simulink model "ROSPiNav2"  (Simulink 10.0)
settings: Solver=FixedStepAuto  StartTime=0.0  StopTime=inf  RelTol=1e-3
libraries: sensehatlib x5, robotlib x2, simulink x1, raspberrypilib x1
settings Model: LogicAnalyzerSignalOrdering=0b4ee2b6-c9ba-4ba2-86b4-30ad931c7907,c8c877dd-a2d7-4449-817a-3d091eaa01f0,b65482df-6083-4df0-8804-932ee4a1c904,d5d3a0d7-9de6-498d-bd3e-b3a3d3b67ba2,3bc10de9-2fa7-4451-9b63-790e2e79518c  Creator=FRED-Surface  LastModifiedBy=FRED-Surface
settings Model: SuppressorTable=|
  | <?xml version="1.0" encoding="UTF-8" standalone="yes" ?>
  | <!DOCTYPE boost_serialization>
  | <boost_serialization signature="serialization::archive" version="15">
  | <DiagnosticSuppressor class_id="0" tracking_level="0" version="6">
  | 	<Table class_id="1" tracking_level="0" version="0">
  | 		<count>1</count>
  | 		<bucket_count>8</bucket_count>
  | 		<item_version>0</item_version>
  | 		<item class_id="2" tracking_level="0" version="0">
  | 			<first class_id="3" tracking_level="0" version="6">
  | 				<Source class_id="4" tracking_level="0" version="0">
  | 					<count>1</count>
  | 					<item_version>0</item_version>
  | 					<item>ROSPiNav2/Counter Limited</item>
  | 				</Source>
  | 			</first>
  | 			<second class_id="5" tracking_level="0" version="6">
  | 				<SuppressedData class_id="6" tracking_level="0" version="0">
  | 					<count>2</count>
  | 					<bucket_count>8</bucket_count>
  | 					<item_version>0</item_version>
  | 					<item class_id="7" tracking_level="0" version="0">
  | 						<first class_id="8" tracking_level="0" version="6">
  | 							<ID>Simulink:DataType:WarningOverFlowDetected</ID>
  | 							<Cause>
  | 								<Source>
  | 									<count>0</count>
  | 									<item_version>0</item_version>
  | 								</Source>
  | 							</Cause>
  | 						</first>
  | 						<second class_id="9" tracking_level="0" version="6">
  | 							<Comment></Comment>
  | 							<User></User>
  | 							<LastModified class_id="10" tracking_level="0" version="0">
  | 								<ptime_date class_id="11" tracking_level="0" version="0">
  | 									<date>20160608</date>
  | 								</ptime_date>
  | 								<ptime_time_duration class_id="12" tracking_level="0" version="0">
  | 									<is_special>0</is_special>
  | 									<time_duration_hours>15</time_duration_hours>
  | 									<time_duration_minutes>23</time_duration_minutes>
  | 									<time_duration_seconds>17</time_duration_seconds>
  | 									<time_duration_fractional_seconds>0</time_duration_fractional_seconds>
  | 								</ptime_time_duration>
  | 							</LastModified>
  | 							<SuppressionType>1</SuppressionType>
  | 						</second>
  | 					</item>
  | 					<item>
  | 						<first>
  | 							<ID>SimulinkFixedPoint:util:Overflowoccurred</ID>
  | 							<Cause>
  | 								<Source>
  | 									<count>0</count>
  | 									<item_version>0</item_version>
  | 								</Source>
  | 							</Cause>
  | 						</first>
  | 						<second>
  | 							<Comment></Comment>
  | 							<User></User>
  | 							<LastModified>
  | 								<ptime_date>
  | 									<date>20160608</date>
  | 								</ptime_date>
  | 								<ptime_time_duration>
  | 									<is_special>0</is_special>
  | 									<time_duration_hours>15</time_duration_hours>
  | 									<time_duration_minutes>23</time_duration_minutes>
  | 									<time_duration_seconds>17</time_duration_seconds>
  | 									<time_duration_fractional_seconds>0</time_duration_fractional_seconds>
  | 								</ptime_time_duration>
  | 							</LastModified>
  | 							<SuppressionType>1</SuppressionType>
  | 						</second>
  | 					</item>
  | 				</SuppressedData>
  | 			</second>
  | 		</item>
  | 	</Table>
  | </DiagnosticSuppressor>
  | </boost_serialization>
settings DataIOCC: SaveFormat=Dataset  ReturnWorkspaceOutputs=on
settings OptimizationCC: EnhancedBackFolding=on  PassReuseOutputArgsAs=Individual arguments  ZeroExternalMemoryAtStartup=off  ZeroInternalMemoryAtStartup=off  LifeSpan=auto  MaxStackSize=64  OptimizeBlockOrder=speed  DifferentSizesBufferReuse=on  OptimizationCustomize=off  EfficientTunableParamExpr=on
settings DebuggingCC: UnderspecifiedInitializationDetection=Simplified  MergeDetectMultiDrivingBlocksExec=error  ParameterTunabilityLossMsg=error  SFUnexpectedBacktrackingDiag=error  SFNoUnconditionalDefaultTransitionDiag=error  SFExecutionAtInitializationDiag=warning  ArithmeticOperatorsInVariantConditions=error
settings HardwareCC: ProdLargestAtomicInteger=Long  ProdLargestAtomicFloat=Double  ProdIntDivRoundTo=Zero  ProdEndianess=LittleEndian  ProdHWDeviceType=ARM Compatible->ARM Cortex
settings ModelReferenceCC: PropagateSignalLabelsOutOfModel=on
settings SFSimCC: SimUseLocalCustomCode=on  MATLABDynamicMemAlloc=off  CustomCodeUndefinedFunction=FilterOut
settings RTWCC: Description=Embedded Coder  SystemTargetFile=ert.tlc  HardwareBoard=Robot Operating System (ROS)  TLCOptions="-aInlineSetEventsForThisBaseRateFcn=TLC_FALSE -aSuppressMultiTaskScheduler=TLC_FALSE  -aRateBasedStepFcn=0"  TemplateMakefile=ert_default_tmf  GenerateReport=on  RTWUseLocalCustomCode=on  Toolchain=Catkin  IncludeHyperlinkInReport=on  LaunchReport=on  TargetLang=C++  GenerateTraceInfo=on  GenerateTraceReport=on  GenerateTraceReportSl=on  GenerateTraceReportSf=on  GenerateTraceReportEml=on
settings MATStruct: className=codertarget.tools.BuildHook  argsTopModelOnly=[]  excludedModels=[]  includeReferencedModels=on  includeTopModel=on  enabled=on  UseCoderTarget=[1]  TargetHardware=Robot Operating System (ROS)  RTOS=Linux  RTOSBaseRateTaskPriority=40  DetectTaskOverruns=[0.0]  Scheduler_interrupt_source=[0.0]  DataVersion=2016.02  IPAddress=ros.codertarget.internal.DeviceParameters.getDeviceAddress  Port=17725  Verbose=[0]  RunInBackground=[1]  Configuration=TCP/IP  MaintainerName=ROS User  MaintainerEmail=rosuser@test.com  License=BSD  DeviceAddress=192.168.0.102  Username=ubuntu  BuildAction=None  Install=/opt/ros/melodic  CatkinWS=~/catkin_ws  ROSTimeStepping=0  ROSTimeNotification=0  StepNotify=/step_notify
settings CodeAppCC: ForceParamTrailComments=on  IgnoreCustomStorageClasses=off  OperatorAnnotations=on  SimulinkDataObjDesc=on  SFDataObjDesc=on  InsertBlockDesc=on  StateflowObjectComments=off
settings ConfigComp: CovMetricSettings=dwe  CovHtmlReporting=off  CovSaveCumulativeToWorkspaceVar=off  CovSaveSingleToWorkspaceVar=off

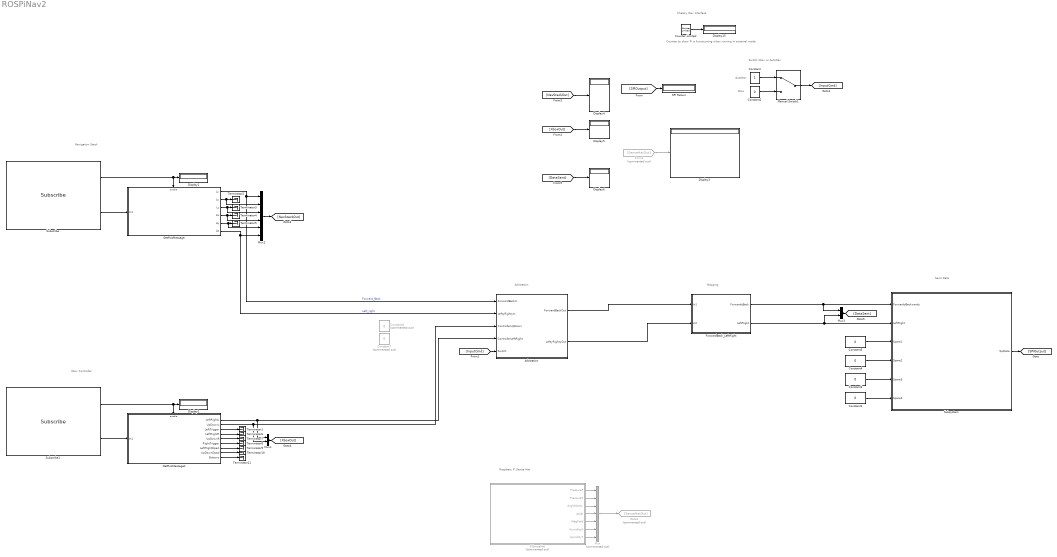
== system ROSPiNav2 ==
  note: Arbitration
  note: Xbox Controller
  note: Raspbery Pi Sense Hat
  note: Switch Xbox or AutoNav
  note: Cheeky Dev Interface
  note: Xbox
  note: Counter to show Pi is functiuoning when running in external mode
  note: Send Data
  note: Navigation Stack
  note: Mapping
  note: AutoNav
  Arbitration : Subsystem
  Constant : Constant  OutDataTypeStr=single
  Constant{1..5} (5 alike) : Constant  Value=0  OutDataTypeStr=single
  Constant6 : Constant  Commented=on  Value=0  OutDataTypeStr=single
  Constant7 : Constant  Commented=on  Value=0  OutDataTypeStr=single
  Counter Limited : simulink/Sources/Counter Limited  uplimit=7  tsamp=1
  Display{1..6,15} (7 alike) : Display
      Display15 settings: Format=bank  Decimation=2
      Display3 settings: Format=bank  Decimation=2
  ForwardBack_LeftRight : Subsystem
  From2 : From  Commented=on  GotoTag=SenseHatOut
  GetRosMessage : Subsystem
  GetRosMessage1 : Subsystem
  Goto2 : Goto  Commented=on  GotoTag=SenseHatOut
  Manual Switch1 : ManualSwitch
  Mux : Mux  Commented=on  Inputs=7
  Mux1 : Mux  Inputs=2
  Mux2 : Mux  Inputs=6
  Mux3 : Mux  Inputs=2
  PiSenseHat : Subsystem  Commented=on
  SPI Return : Display
      settings: Format=bank  Decimation=2
  Subscribe : robotlib/Subscribe  topicSource=Select from ROS network  topic=/planner/cmd_vel  messageType=geometry_msgs/Twist  sampleTime=0.1  messageQueueLength=1
      settings: SourceProductName=ROS Toolbox
  Subscribe1 : robotlib/Subscribe  topicSource=Specify your own  topic=/joy  messageType=sensor_msgs/Joy  sampleTime=0.1  messageQueueLength=1
      settings: SourceProductName=ROS Toolbox
  Subsystem : Subsystem
  Terminator{1..11} (11 alike) : Terminator
  wires:
  GetRosMessage1/2(UpDownL) -> Mux1/2, Arbitration/3("ControllerUpDown ")
  [SPIOutput] -> SPI Return/1
  Mux3/1 -> [DataSent]
  [DataSent] -> Display6/1
  [InputCmd] -> Arbitration/5("Switch ")
  GetRosMessage1/9("Buttons ") -> Terminator11/1
  Constant5/1 -> Subsystem/3(Spare1)
  GetRosMessage1/7(LeftRightDpad) -> Terminator9/1
  Constant4/1 -> Subsystem/4(Spare2)
  Constant/1 -> Manual Switch1/1
  ForwardBack_LeftRight/1(ForwardsBack) -> Mux3/1, Subsystem/1(ForwardsBackwards)
  ForwardBack_LeftRight/2(LeftRight) -> Mux3/2, Subsystem/2(LeftRight)
  GetRosMessage1/5(UpDownR) -> Terminator7/1
  Arbitration/1(ForwardBackOut) -> ForwardBack_LeftRight/1(In1)
  Subscribe/2 -> GetRosMessage/1(In1)
  GetRosMessage/5("Ay ") -> Mux2/5, Terminator5/1
  GetRosMessage/3(Lz) -> Mux2/3, Terminator3/1
  Constant2/1 -> Manual Switch1/2
  GetRosMessage/4(Ax) -> Mux2/4, Terminator4/1
  GetRosMessage1/4(LeftRightR) -> Terminator6/1
  PiSenseHat/1(PressureP) -> Mux/1
  From2/1 -> Display3/1
  Subscribe/1 -> GetRosMessage/Enable, Display1/1
  GetRosMessage/2("Ly ") -> Mux2/2, Terminator2/1
  Subscribe1/2 -> GetRosMessage1/1(In1)
  [XboxOut] -> Display5/1
  PiSenseHat/7(HumidityT) -> Mux/7
  Constant3/1 -> Subsystem/5(Spare3)
  GetRosMessage1/8(UpDownDpad) -> Terminator10/1
  Mux2/1 -> [NavStackOut]
  Subscribe1/1 -> GetRosMessage1/Enable, Display2/1
  GetRosMessage/6("Az ") -> Arbitration/2(LeftyRightyIn), Mux2/6  "Left_right"
  PiSenseHat/5(MagField) -> Mux/5
  Subsystem/1(SpiData) -> [SPIOutput]
  Constant1/1 -> Subsystem/6(Spare4)
  Mux1/1 -> [XboxOut]
  PiSenseHat/4(Accel) -> Mux/4
  Counter Limited/1 -> Display15/1
  GetRosMessage1/1(LeftRightL) -> Mux1/1, Arbitration/4(ControllerLeftRight)
  GetRosMessage1/3(LeftTrigger) -> Terminator1/1
  GetRosMessage1/6(RightTrigger) -> Terminator8/1
  Arbitration/2(LeftyRightyOut) -> ForwardBack_LeftRight/2(In2)
  GetRosMessage/1(Lx) -> Mux2/1, Arbitration/1(ForwardBackIn)  "Forward_Back"
  [NavStackOut] -> Display4/1
  Manual Switch1/1 -> [InputCmd]
  PiSenseHat/3(AngVelocity) -> Mux/3
  Mux/1 -> Goto2/1
  PiSenseHat/6(HumidityH) -> Mux/6
  PiSenseHat/2(PressureT) -> Mux/2

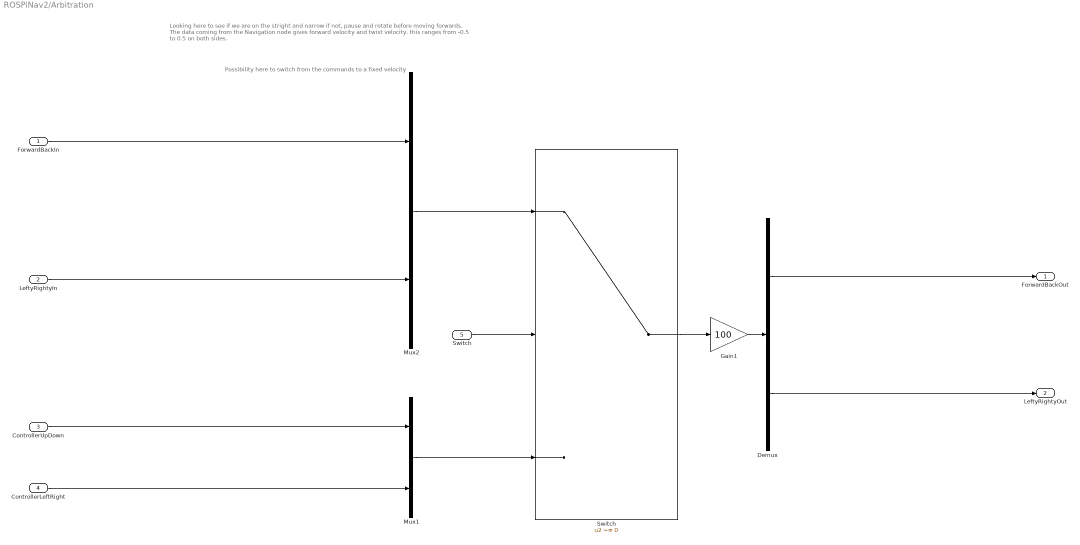
== system ROSPiNav2/Arbitration ==
  note: Possibility here to switch from the commands to a fixed velocity
  note: Looking here to see if we are on the stright and narrow if not, pause and rotate before moving forwards.
      | The data coming from the Navigation node gives forward velocity and twist velocity. this ranges from -0.5 to 0.5 on both sides.
  ForwardBackIn : Inport
  LeftyRightyIn : Inport  Port=2
  "ControllerUpDown " : Inport  Port=3
  ControllerLeftRight : Inport  Port=4
  "Switch " : Inport  Port=5
  Demux : Demux  Outputs=2
  Gain1 : Gain  Gain=100
  Mux1 : Mux  Inputs=2
  Mux2 : Mux  Inputs=2
  Switch : Switch  Criteria=u2 ~= 0
  ForwardBackOut : Outport
  LeftyRightyOut : Outport  Port=2
  wires:
  LeftyRightyIn/1 -> Mux2/2
  Demux/1 -> ForwardBackOut/1
  Demux/2 -> LeftyRightyOut/1
  Switch/1 -> Gain1/1
  "ControllerUpDown "/1 -> Mux1/1
  ControllerLeftRight/1 -> Mux1/2
  Mux1/1 -> Switch/3
  "Switch "/1 -> Switch/2
  Gain1/1 -> Demux/1
  Mux2/1 -> Switch/1
  ForwardBackIn/1 -> Mux2/1

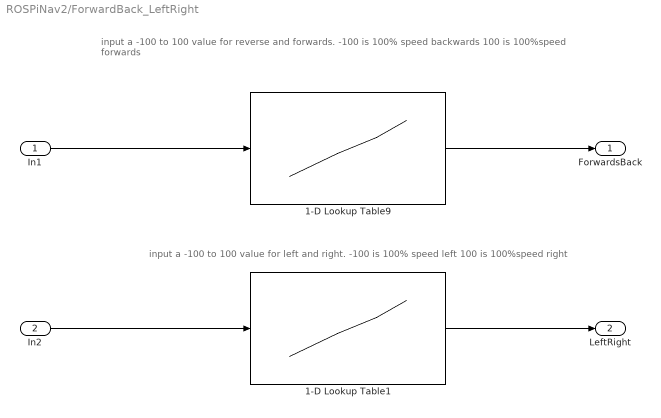
== system ROSPiNav2/ForwardBack_LeftRight ==
  note: input a -100 to 100 value for reverse and forwards. -100 is 100% speed backwards 100 is 100%speed forwards
  note: input a -100 to 100 value for left and right. -100 is 100% speed left 100 is 100%speed right
  In1 : Inport
  In2 : Inport  Port=2
  1-D Lookup Table1 : Lookup_n-D  NumberOfTableDimensions=1  BreakpointsForDimension1=[-100,-50,0,50,100]  BreakpointsForDimension1FirstPoint=0  BreakpointsForDimension1Spacing=1.8  Table=[1000;1250;1500;1750;2000;]  ExtrapMethod=Clip  InternalRulePriority=Speed  OutDataTypeStr=single  RndMeth=Simplest  InputSameDT=on
  1-D Lookup Table9 : Lookup_n-D  NumberOfTableDimensions=1  BreakpointsForDimension1=[-100,-50,0,50,100]  BreakpointsForDimension1FirstPoint=0  BreakpointsForDimension1Spacing=1.8  Table=[1000;1250;1500;1750;2000]  ExtrapMethod=Clip  InternalRulePriority=Speed  OutDataTypeStr=single  RndMeth=Simplest  InputSameDT=on
  ForwardsBack : Outport  OutDataTypeStr=single
  LeftRight : Outport  Port=2  OutDataTypeStr=single
  wires:
  In1/1 -> 1-D Lookup Table9/1
  1-D Lookup Table1/1 -> LeftRight/1
  1-D Lookup Table9/1 -> ForwardsBack/1
  In2/1 -> 1-D Lookup Table1/1

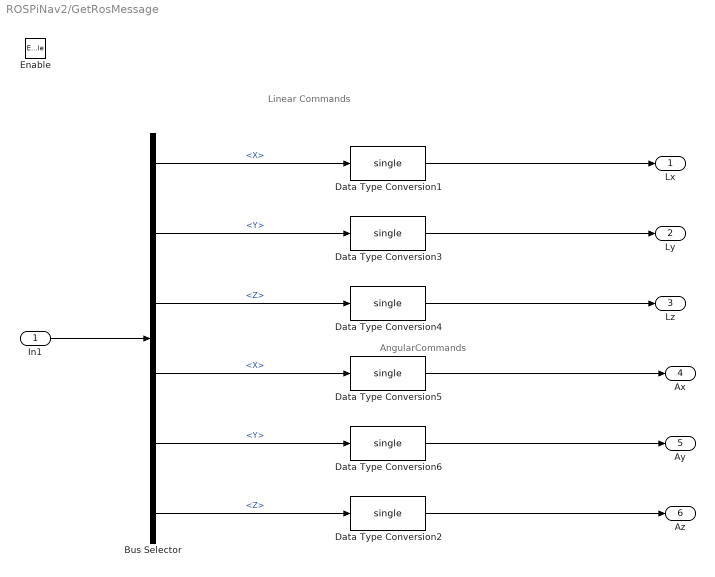
== system ROSPiNav2/GetRosMessage ==
  note: Linear Commands
  note: AngularCommands
  In1 : Inport
  Enable : EnablePort
  Bus Selector : BusSelector  OutputSignals=Linear.X,Linear.Y,Linear.Z,Angular.X,Angular.Y,Angular.Z
  Data Type Conversion{1..6} (6 alike) : DataTypeConversion  OutDataTypeStr=single
  Lx : Outport  OutDataTypeStr=single
  "Ly " : Outport  Port=2
  Lz : Outport  Port=3
  Ax : Outport  Port=4
  "Ay " : Outport  Port=5
  "Az " : Outport  Port=6  OutDataTypeStr=single
  wires:
  Bus Selector/2 -> Data Type Conversion3/1  "<Y>"
  Bus Selector/1 -> Data Type Conversion1/1  "<X>"
  In1/1 -> Bus Selector/1
  Bus Selector/3 -> Data Type Conversion4/1  "<Z>"
  Bus Selector/4 -> Data Type Conversion5/1  "<X>"
  Bus Selector/5 -> Data Type Conversion6/1  "<Y>"
  Bus Selector/6 -> Data Type Conversion2/1  "<Z>"
  Data Type Conversion1/1 -> Lx/1
  Data Type Conversion2/1 -> "Az "/1
  Data Type Conversion3/1 -> "Ly "/1
  Data Type Conversion4/1 -> Lz/1
  Data Type Conversion5/1 -> Ax/1
  Data Type Conversion6/1 -> "Ay "/1

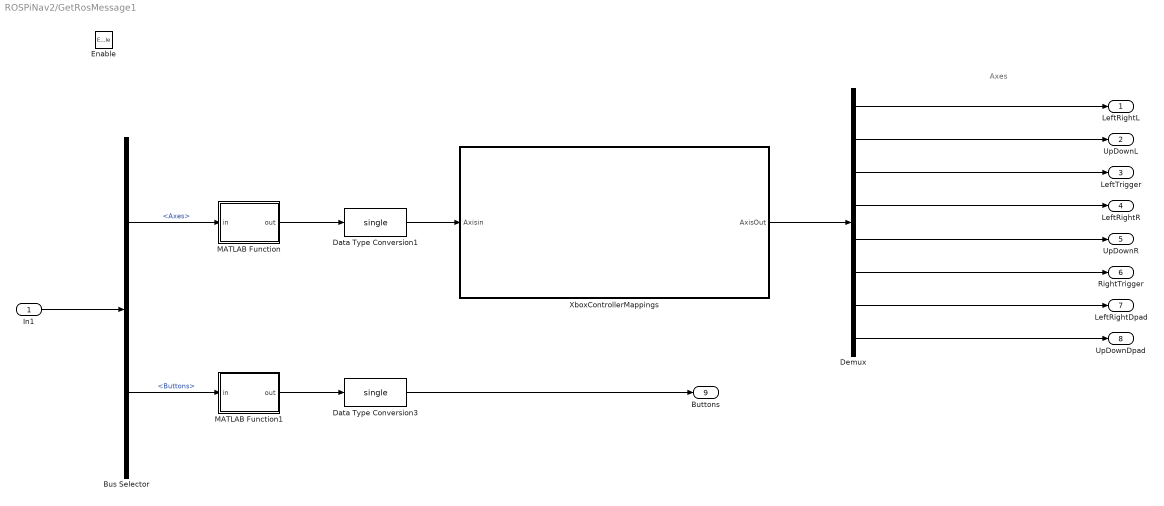
== system ROSPiNav2/GetRosMessage1 ==
  note: Axes
  In1 : Inport
  Enable : EnablePort
  Bus Selector : BusSelector  OutputSignals=Axes,Buttons
  Data Type Conversion1 : DataTypeConversion  OutDataTypeStr=single
  Data Type Conversion3 : DataTypeConversion  OutDataTypeStr=single
  Demux : Demux  Outputs=8
  MATLAB Function : MATLAB Function  TreatAsAtomicUnit=on
  MATLAB Function1 : MATLAB Function  TreatAsAtomicUnit=on
  "XboxControllerMappings " : Subsystem
  LeftRightL : Outport  OutDataTypeStr=single
  UpDownL : Outport  Port=2  OutDataTypeStr=single
  LeftTrigger : Outport  Port=3  OutDataTypeStr=single
  LeftRightR : Outport  Port=4  OutDataTypeStr=single
  UpDownR : Outport  Port=5  OutDataTypeStr=single
  RightTrigger : Outport  Port=6  OutDataTypeStr=single
  LeftRightDpad : Outport  Port=7  OutDataTypeStr=single
  UpDownDpad : Outport  Port=8  OutDataTypeStr=single
  "Buttons " : Outport  Port=9
  wires:
  Data Type Conversion3/1 -> "Buttons "/1
  Demux/1 -> LeftRightL/1
  In1/1 -> Bus Selector/1
  Bus Selector/1 -> MATLAB Function/1(in)  "<Axes>"
  Bus Selector/2 -> MATLAB Function1/1(in)  "<Buttons>"
  Data Type Conversion1/1 -> "XboxControllerMappings "/1(Axisin)
  Demux/2 -> UpDownL/1
  Demux/3 -> LeftTrigger/1
  Demux/4 -> LeftRightR/1
  Demux/5 -> UpDownR/1
  Demux/6 -> RightTrigger/1
  Demux/7 -> LeftRightDpad/1
  "XboxControllerMappings "/1(AxisOut) -> Demux/1
  Demux/8 -> UpDownDpad/1
  MATLAB Function/1(out) -> Data Type Conversion1/1
  MATLAB Function1/1(out) -> Data Type Conversion3/1

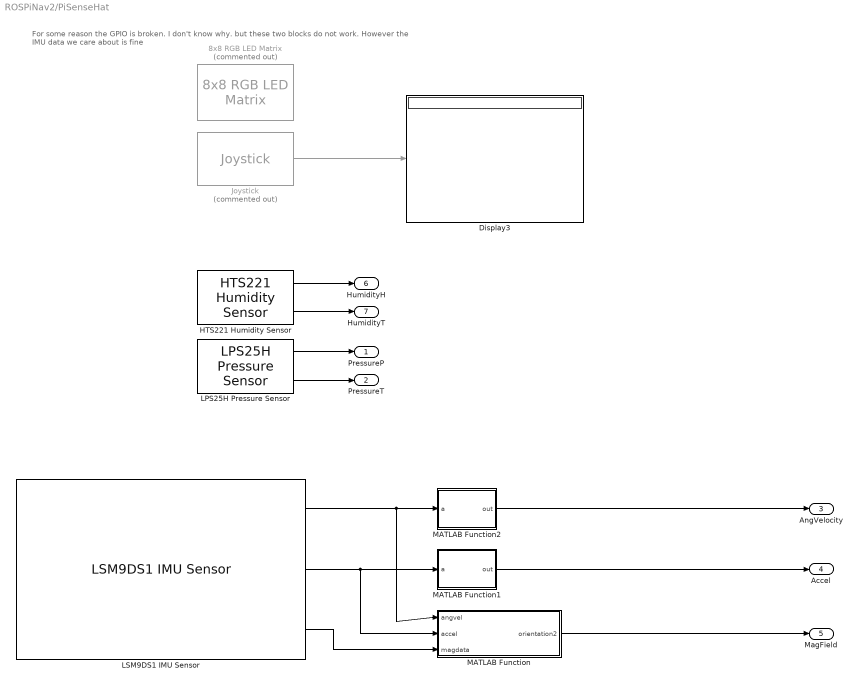
== system ROSPiNav2/PiSenseHat ==
  note: For some reason the GPIO is broken. I don't know why. but these two blocks do not work. However the IMU data we care about is fine
  "8x8 RGB LED Matrix " : sensehatlib/8x8 RGB LED Matrix   Commented=on  Mode=Write Pixel  ImageSource=One multidimensional signal  OrientationSource=Block dialog  LEDOrientation=0  blockPlatform=Raspberry pi
      settings: SourceProductName=Simulink Support Package for Raspberry Pi Hardware  SourceProductBaseCode=RASPPI
  Display3 : Display
      settings: Format=bank  Decimation=2
  HTS221 Humidity Sensor : sensehatlib/HTS221 Humidity Sensor  BoardProperty=Pi 2 Model B  OutputDataRate=12.5 Hz  SampleTime=0.1
      settings: SourceProductName=Simulink Support Package for Raspberry Pi Hardware  SourceProductBaseCode=RASPPI
  Joystick : sensehatlib/Joystick  Commented=on  SampleTime=0.5  blockPlatform=Raspberry Pi
      settings: SourceProductName=Simulink Support Package for Raspberry Pi Hardware  SourceProductBaseCode=RASPPI
  LPS25H Pressure Sensor : sensehatlib/LPS25H Pressure Sensor  BoardProperty=Pi 3 Model B+  OutputDataRate=12.5 Hz  SampleTime=0.2
      settings: SourceProductName=Simulink Support Package for Raspberry Pi Hardware  SourceProductBaseCode=RASPPI
  LSM9DS1 IMU Sensor : sensehatlib/LSM9DS1 IMU Sensor  blockPlatform=Raspberry Pi  BoardProperty_sh=Pi 3 Model B  ActiveSensors_=Accelerometer, Gyroscope and Magnetometer  AccelerometerOutputDataRate=119 Hz  AccelerometerFullScaleRange=+/- 2g  AccelerometerBandwidth=50 Hz  GyroscopeOutputDataRate=119 Hz  GyroscopeFullScaleRange=245 dps  GyroscopeBandwidthMode=0  GyroscopeHighPassFilterEnabled=off  GyroscopeHighPassFilterMode=0  MagnetometerFullScaleRange=+/- 4 gauss  MagnetometerOutputDataRate=40 Hz  SampleTime=0.1
      settings: SourceProductName=Simulink Support Package for Raspberry Pi Hardware  SourceProductBaseCode=RASPPI
  MATLAB Function : MATLAB Function  TreatAsAtomicUnit=on
  MATLAB Function1 : MATLAB Function  TreatAsAtomicUnit=on
  MATLAB Function2 : MATLAB Function  TreatAsAtomicUnit=on
  PressureP : Outport
  PressureT : Outport  Port=2
  AngVelocity : Outport  Port=3
  Accel : Outport  Port=4
  MagField : Outport  Port=5
  HumidityH : Outport  Port=6
  HumidityT : Outport  Port=7
  wires:
  HTS221 Humidity Sensor/2 -> HumidityT/1
  HTS221 Humidity Sensor/1 -> HumidityH/1
  Joystick/1 -> Display3/1
  LSM9DS1 IMU Sensor/1 -> MATLAB Function/1(angvel), MATLAB Function2/1(a)
  LPS25H Pressure Sensor/1 -> PressureP/1
  LPS25H Pressure Sensor/2 -> PressureT/1
  LSM9DS1 IMU Sensor/2 -> MATLAB Function/2(accel), MATLAB Function1/1(a)
  MATLAB Function/1(orientation2) -> MagField/1
  MATLAB Function1/1(out) -> Accel/1
  MATLAB Function2/1(out) -> AngVelocity/1
  LSM9DS1 IMU Sensor/3 -> MATLAB Function/3(magdata)

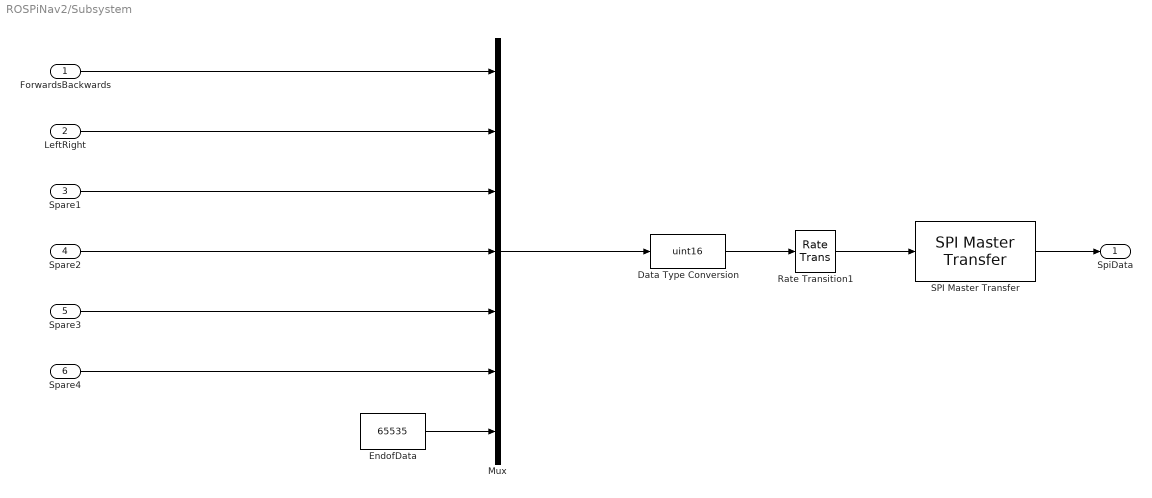
== system ROSPiNav2/Subsystem ==
  ForwardsBackwards : Inport
  LeftRight : Inport  Port=2
  Spare1 : Inport  Port=3
  Spare2 : Inport  Port=4
  Spare3 : Inport  Port=5
  Spare4 : Inport  Port=6
  Data Type Conversion : DataTypeConversion  OutDataTypeStr=uint16  RndMeth=Round  SaturateOnIntegerOverflow=on
  EndofData : Constant  Value=65535  OutDataTypeStr=single
  Mux : Mux  Inputs=7
  Rate Transition1 : RateTransition  OutPortSampleTime=0.1
  SPI Master Transfer : raspberrypilib/SPI Master Transfer  BoardProperty=Pi 3 Model B+  SPIModule=uint32(0)  Mode=Master  BusSpeed=1000000  Pin=SPI0_CE0  FirstBitToTransfer=Most significant bit (MSB)  ClockMode=0  BlockFunction=Transfer  RegisterAddress=0  OutputDataType=int8  OutputDataLength=1
      settings: SourceProductName=Simulink Support Package for Raspberry Pi Hardware  SourceProductBaseCode=RASPPI
  SpiData : Outport
  wires:
  LeftRight/1 -> Mux/2
  ForwardsBackwards/1 -> Mux/1
  Spare4/1 -> Mux/6
  Mux/1 -> Data Type Conversion/1
  EndofData/1 -> Mux/7
  Rate Transition1/1 -> SPI Master Transfer/1
  Data Type Conversion/1 -> Rate Transition1/1
  Spare2/1 -> Mux/4
  Spare3/1 -> Mux/5
  SPI Master Transfer/1 -> SpiData/1
  Spare1/1 -> Mux/3

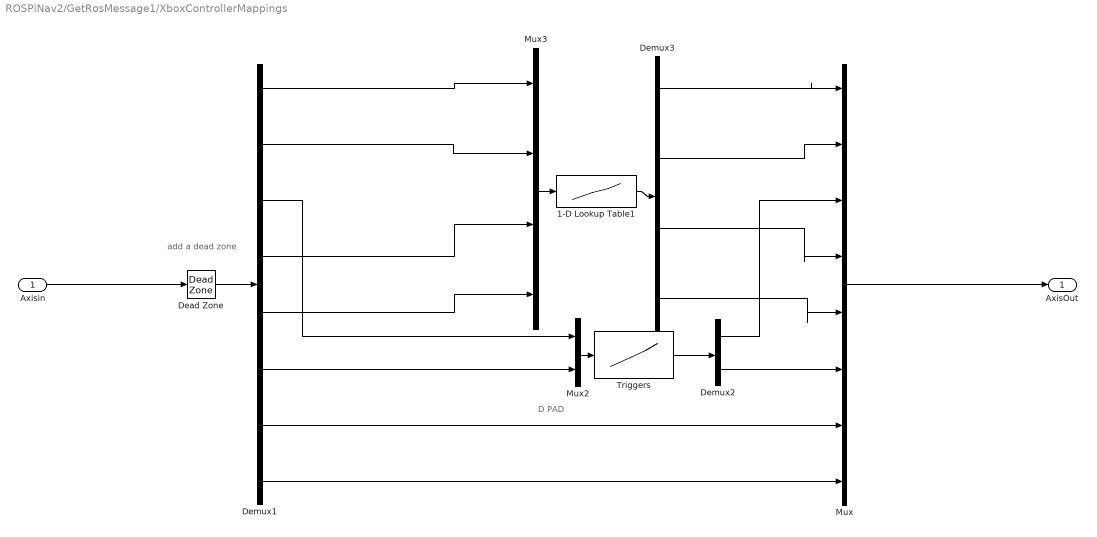
== system ROSPiNav2/GetRosMessage1/XboxControllerMappings  ==
  note: add a dead zone
  note: D PAD
  Axisin : Inport
  1-D Lookup Table1 : Lookup_n-D  NumberOfTableDimensions=1  BreakpointsForDimension1=[-0.9,0,0.9]  Table=[-1,0,1]  InternalRulePriority=Speed  RndMeth=Simplest  InputSameDT=on
  Dead Zone : DeadZone  LowerValue=-0.1  UpperValue=0.1  SaturateOnIntegerOverflow=on
  Demux1 : Demux  Outputs=8
  Demux2 : Demux  Outputs=2
  Demux3 : Demux
  Mux : Mux  Inputs=8
  Mux2 : Mux  Inputs=2
  Mux3 : Mux
  Triggers : Lookup_n-D  NumberOfTableDimensions=1  BreakpointsForDimension1=[-0.9,0,0.9]  Table=[0,0.5,1]  InternalRulePriority=Speed  RndMeth=Simplest  InputSameDT=on
  AxisOut : Outport
  wires:
  Demux1/2 -> Mux3/2
  Demux1/3 -> Mux2/1
  Demux1/1 -> Mux3/1
  Demux1/7 -> Mux/7
  Axisin/1 -> Dead Zone/1
  Demux1/5 -> Mux3/4
  Demux1/6 -> Mux2/2
  Demux1/8 -> Mux/8
  Mux3/1 -> 1-D Lookup Table1/1
  Dead Zone/1 -> Demux1/1
  Demux1/4 -> Mux3/3
  Triggers/1 -> Demux2/1
  Mux2/1 -> Triggers/1
  Mux/1 -> AxisOut/1
  1-D Lookup Table1/1 -> Demux3/1
  Demux2/2 -> Mux/6
  Demux2/1 -> Mux/3
  Demux3/1 -> Mux/1
  Demux3/2 -> Mux/2
  Demux3/3 -> Mux/4
  Demux3/4 -> Mux/5

== matlab function GetRosMessage1/MATLAB Function1 ==
  data: in input double; out output double
function out = fcn(in)

out = in(1:7);

== matlab function GetRosMessage1/MATLAB Function ==
  data: in input double; out output double
function out = fcn(in)

out = in(1:8);

== matlab function PiSenseHat/MATLAB Function ==
  data: angvel input double; orientation2 output double; accel input double; magdata input double
function orientation2 = fcn(angvel, accel, magdata)

% x = a(:,1);
% y = a(:,2);
% z = a(:,3);
decim = 1;
FUSE = ahrsfilter('DecimationFactor',decim);
% out = atan(y/x) * (180/pi);
% orientation = 0;
[orientation] = FUSE(accel,angvel,magdata);
orientation = eulerd(orientation,'ZYX','frame');
orientation2 = orientation(1,3);

== matlab function PiSenseHat/MATLAB Function1 ==
  data: a input double; out output double
function out = fcn(a)
x = a(:,1);
y = a(:,2);
z = a(:,3);
out = sqrt(sum(x.^2 + y.^2 + z.^2, 2));

== matlab function PiSenseHat/MATLAB Function2 ==
  data: a input double; out output double
function out = fcn(a)
x = a(:,1);
y = a(:,2);
z = a(:,3);
out = sqrt(sum(x.^2 + y.^2 + z.^2, 2));
